simulink model "Lab6_pid_ciagly"  (R2017a)
settings: Solver=VariableStepAuto  StartTime=0.0  StopTime=10.0  MaxStep=0.01  RelTol=1e-3
libraries: cstblocks x2
settings Model: Creator=ishiguro  LastModifiedBy=ishiguro
settings DataIOCC: TimeSaveName=tout_PID_ciagly

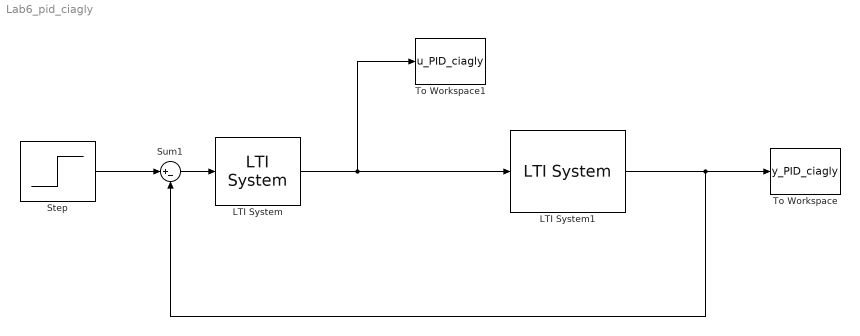
== system Lab6_pid_ciagly ==
  LTI System : cstblocks/LTI System  sys=Kr_pid  IC=[]
  LTI System1 : cstblocks/LTI System  sys=K  IC=[]
  Step : Step  Time=0  SampleTime=0
  Sum1 : Sum  Inputs=|+-
  To Workspace : ToWorkspace  VariableName=y_PID_ciagly  SampleTime=-1
  To Workspace1 : ToWorkspace  VariableName=u_PID_ciagly  SampleTime=-1
  wires:
  Step/1 -> Sum1/1
  Sum1/1 -> LTI System/1
  LTI System/1 -> LTI System1/1, To Workspace1/1
  LTI System1/1 -> Sum1/2, To Workspace/1
